simulink model "Simulation"  (R2023b)
settings: Solver=VariableStepAuto  StartTime=0.0  StopTime=2  RelTol=1e-3
InitFcn:
  | Tsc=0.0001;
  | Rs=0.0113929;
  | Rr=0.0197883;
  | Ls=0.007145;
  | Lr=0.007145;
  | Lm=0.007045;
  | w_c=100;
libraries: slpidlib x6, simulink x1, spspowerguiLib x1
(part 2 of 2)

== matlab function Simulation/MATLAB Function1 ==
  data: phir_vm_alpha input; Theta output; phir_vm_beta input
function Theta = Flux(phir_vm_alpha,phir_vm_beta)
theta=double(atan2(phir_vm_beta,phir_vm_alpha));
theta=theta+2*pi;
%%
if theta>2*pi
   theta=theta-2*pi;
end
Theta=double(theta);
end
